simulink model "CP_SFC_Lin_a_n9945008"  (R2018b)
settings: Solver=ode4  StartTime=0.0  StopTime=5  FixedStep=0.02  RelTol=1e-3
values from neighbouring files (symbols this model uses):
  Aa = [ 0 ,       0            , 1 , 0 ... (first row only)    [CP_SFC_Lin_a_MainFile_n9945008.m]
  Ba = [0;0;1/Mc;-1/(l*Mc)]    [CP_SFC_Lin_a_MainFile_n9945008.m]
  Ca = eye(4)    [CP_SFC_Lin_a_MainFile_n9945008.m]
  Da = zeros(4,1)    [CP_SFC_Lin_a_MainFile_n9945008.m]
  Ka = place(Aa,Ba, [-3,-4,-5,-6])    [CP_SFC_Lin_a_MainFile_n9945008.m]
  x0 = [0.2 20*pi/180 0 0]'    [CP_SFC_Lin_a_MainFile_n9945008.m]    (also in CP_SFC_Lin_b_MainFile_n9945008.m = [0.4 200*pi/180 0 0]')
settings Model: Creator=Cody  LastModifiedBy=Cody

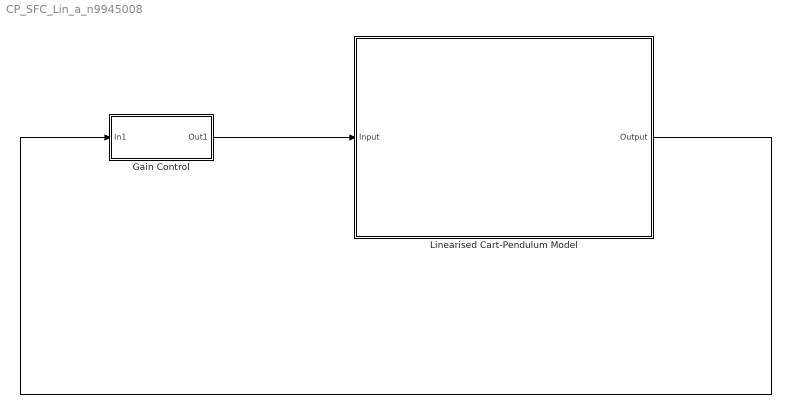
== system CP_SFC_Lin_a_n9945008 ==
  Gain Control : Subsystem
  "Linearised Cart-Pendulum Model " : Subsystem
  wires:
  Gain Control/1(Out1) -> "Linearised Cart-Pendulum Model "/1(Input)
  "Linearised Cart-Pendulum Model "/1(Output) -> Gain Control/1(In1)

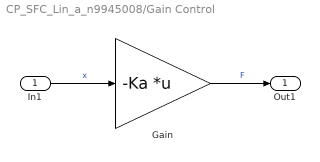
== system CP_SFC_Lin_a_n9945008/Gain Control ==
  In1 : Inport
  Gain : Gain  Gain=-Ka  Multiplication=Matrix(K*u)
  Out1 : Outport
  wires:
  In1/1 -> Gain/1  "x"
  Gain/1 -> Out1/1  "F"

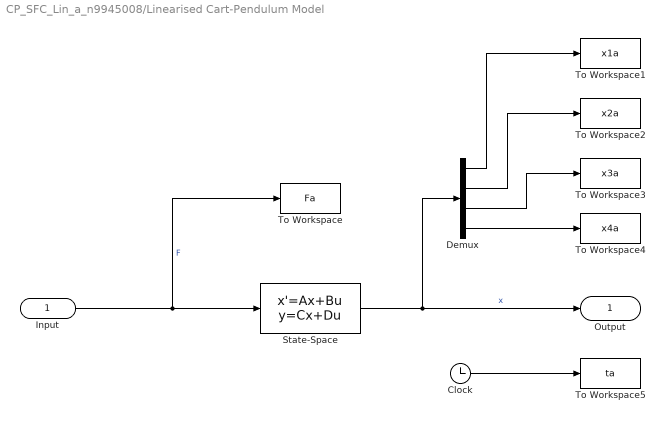
== system CP_SFC_Lin_a_n9945008/Linearised Cart-Pendulum Model  ==
  Input : Inport
  Clock : Clock
  Demux : Demux
  State-Space : StateSpace  A=Aa  B=Ba  C=Ca  D=Da  InitialCondition=x0
  To Workspace : ToWorkspace  VariableName=Fa  SampleTime=-1
      settings: Save2DSignal=2-D array (concatenate along first dimension)
  To Workspace1 : ToWorkspace  VariableName=x1a  SampleTime=-1
      settings: Save2DSignal=2-D array (concatenate along first dimension)
  To Workspace2 : ToWorkspace  VariableName=x2a  SampleTime=-1
      settings: Save2DSignal=2-D array (concatenate along first dimension)
  To Workspace3 : ToWorkspace  VariableName=x3a  SampleTime=-1
      settings: Save2DSignal=2-D array (concatenate along first dimension)
  To Workspace4 : ToWorkspace  VariableName=x4a  SampleTime=-1
      settings: Save2DSignal=2-D array (concatenate along first dimension)
  To Workspace5 : ToWorkspace  VariableName=ta  SampleTime=-1
      settings: Save2DSignal=2-D array (concatenate along first dimension)
  Output : Outport
  wires:
  Clock/1 -> To Workspace5/1
  Demux/1 -> To Workspace1/1
  State-Space/1 -> Demux/1, Output/1  "x"
  Demux/4 -> To Workspace4/1
  Input/1 -> To Workspace/1, State-Space/1  "F"
  Demux/2 -> To Workspace2/1
  Demux/3 -> To Workspace3/1
